simulink model "hw3Task4"  (R2020a)
settings: Solver=VariableStepAuto  StartTime=0.0  StopTime=10  MaxStep=0.01  RelTol=1e-4  EnableMultiTasking=on
libraries: simulink x2
settings Model: Creator=polinaturiseva  LastModifiedBy=polinaturiseva
settings DataIOCC: LimitDataPoints=on  SaveOutput=off  SaveTime=off
settings OptimizationCC: ExpressionDepthLimit=2147483647  LifeSpan=1
settings DebuggingCC: UnderspecifiedInitializationDetection=Classic  MergeDetectMultiDrivingBlocksExec=none  FcnCallInpInsideContextMsg=warning  AllowSymbolicDim=off  StateNameClashWarn=warning  SFUnexpectedBacktrackingDiag=warning  SFNoUnconditionalDefaultTransitionDiag=warning  SFExecutionAtInitializationDiag=none  ArithmeticOperatorsInVariantConditions=warning
settings SFSimCC: SimUseLocalCustomCode=off  CustomCodeUndefinedFunction=UseInterfaceOnly
settings RTWCC: RTWUseLocalCustomCode=off
settings CodeAppCC: StateflowObjectComments=on
settings GRTTargetCC: TargetLangStandard=C89/C90 (ANSI)  CombineOutputUpdateFcns=off  GRTInterface=on

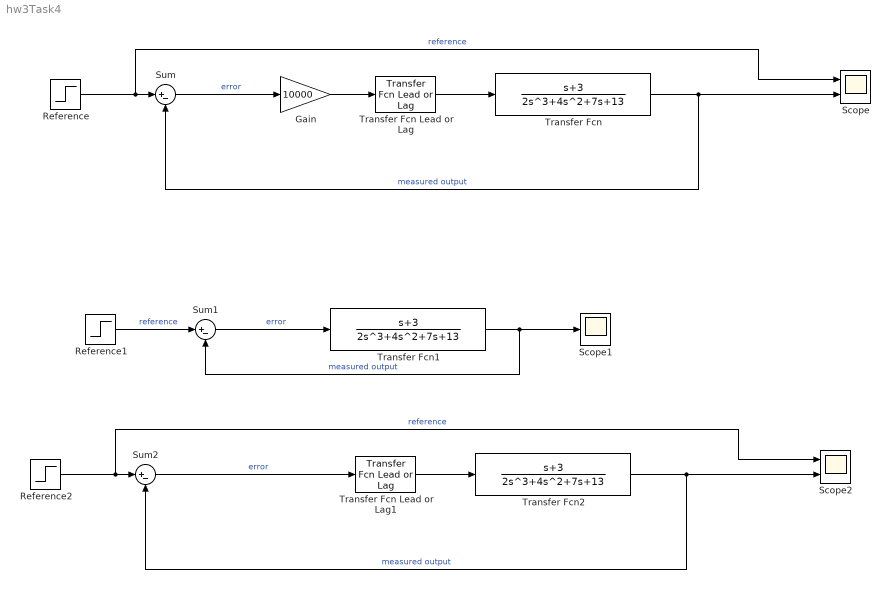
== system hw3Task4 ==
  Gain : Gain  Gain=10000
  Reference : Step  SampleTime=0
  Reference1 : Step  SampleTime=0
  Reference2 : Step  SampleTime=0
  Scope : Scope  NumInputPorts=2
  Scope1 : Scope
  Scope2 : Scope  NumInputPorts=2
  Sum : Sum  Inputs=|+-
  Sum1 : Sum  Inputs=|+-
  Sum2 : Sum  Inputs=|+-
  Transfer Fcn : TransferFcn  Numerator=[1 3]  Denominator=[2 4 7 13]
  Transfer Fcn Lead or Lag : simulink/Discrete/Transfer Fcn Lead or Lag  PoleZ=0.01  ZeroZ=0.9  ICPrevOutput=0.0  ICPrevInput=0.0  DoSatur=off
      settings: SourceProductBaseCode=SL
  Transfer Fcn Lead or Lag1 : simulink/Discrete/Transfer Fcn Lead or Lag  PoleZ=0.1  ZeroZ=0.9  ICPrevOutput=0.0  ICPrevInput=0.0  DoSatur=off
      settings: SourceProductBaseCode=SL
  Transfer Fcn1 : TransferFcn  Numerator=[1 3]  Denominator=[2 4 7 13]
  Transfer Fcn2 : TransferFcn  Numerator=[1 3]  Denominator=[2 4 7 13]
  wires:
  Reference/1 -> Scope/1, Sum/1  "reference"
  Transfer Fcn/1 -> Sum/2, Scope/2  "measured output"
  Sum/1 -> Gain/1  "error"
  Transfer Fcn Lead or Lag/1 -> Transfer Fcn/1
  Gain/1 -> Transfer Fcn Lead or Lag/1
  Reference1/1 -> Sum1/1  "reference"
  Transfer Fcn1/1 -> Sum1/2, Scope1/1  "measured output"
  Sum1/1 -> Transfer Fcn1/1  "error"
  Sum2/1 -> Transfer Fcn Lead or Lag1/1  "error"
  Transfer Fcn Lead or Lag1/1 -> Transfer Fcn2/1
  Reference2/1 -> Scope2/1, Sum2/1  "reference"
  Transfer Fcn2/1 -> Sum2/2, Scope2/2  "measured output"
